simulink model "TST_CoVMD_TrqDesCoord"  (R2016b)
settings: Solver=FixedStepDiscrete  StartTime=0.0  StopTime=simTime  FixedStep=sampleTime  RelTol=1e-3
values from neighbouring files (symbols this model uses):
  testCase = 1    [initTST_CoVMD_TrqDesCoord_001.m]
libraries: simulink x12, UnitTest_Lib x10
settings Model: Creator=zhengjinyan  LastModifiedBy=zhengjinyan
settings DebuggingCC: SignalRangeChecking=error

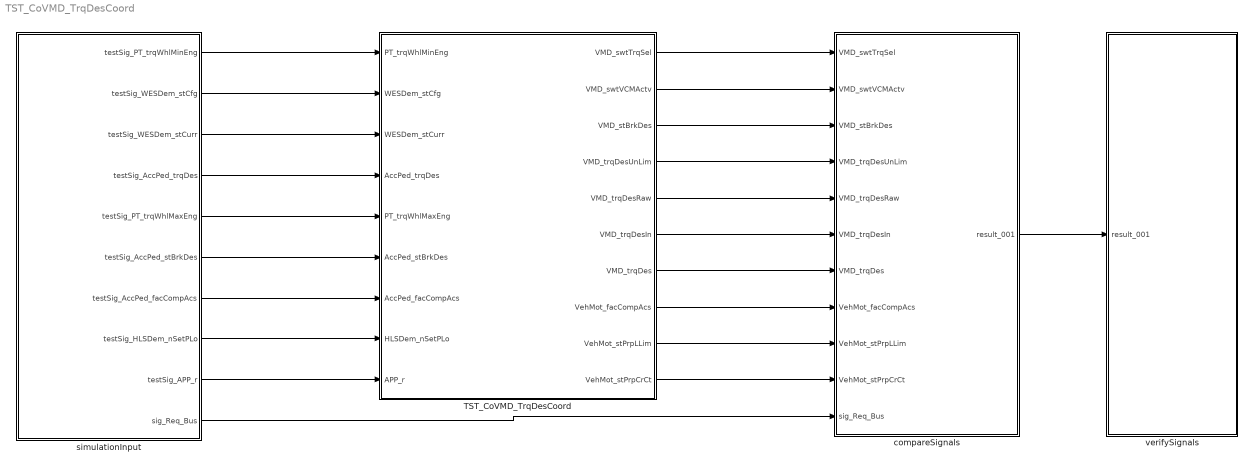
== system TST_CoVMD_TrqDesCoord ==
  TST_CoVMD_TrqDesCoord : Subsystem
  compareSignals : Subsystem
  simulationInput : Subsystem
  verifySignals : Subsystem
  wires:
  simulationInput/1(testSig_PT_trqWhlMinEng) -> TST_CoVMD_TrqDesCoord/1(PT_trqWhlMinEng)
  simulationInput/2(testSig_WESDem_stCfg) -> TST_CoVMD_TrqDesCoord/2(WESDem_stCfg)
  simulationInput/3(testSig_WESDem_stCurr) -> TST_CoVMD_TrqDesCoord/3(WESDem_stCurr)
  simulationInput/4(testSig_AccPed_trqDes) -> TST_CoVMD_TrqDesCoord/4(AccPed_trqDes)
  simulationInput/5(testSig_PT_trqWhlMaxEng) -> TST_CoVMD_TrqDesCoord/5(PT_trqWhlMaxEng)
  simulationInput/6(testSig_AccPed_stBrkDes) -> TST_CoVMD_TrqDesCoord/6(AccPed_stBrkDes)
  simulationInput/7(testSig_AccPed_facCompAcs) -> TST_CoVMD_TrqDesCoord/7(AccPed_facCompAcs)
  simulationInput/8(testSig_HLSDem_nSetPLo) -> TST_CoVMD_TrqDesCoord/8(HLSDem_nSetPLo)
  simulationInput/9(testSig_APP_r) -> TST_CoVMD_TrqDesCoord/9(APP_r)
  TST_CoVMD_TrqDesCoord/1(VMD_swtTrqSel) -> compareSignals/1(VMD_swtTrqSel)
  TST_CoVMD_TrqDesCoord/2(VMD_swtVCMActv) -> compareSignals/2(VMD_swtVCMActv)
  TST_CoVMD_TrqDesCoord/3(VMD_stBrkDes) -> compareSignals/3(VMD_stBrkDes)
  TST_CoVMD_TrqDesCoord/4(VMD_trqDesUnLim) -> compareSignals/4(VMD_trqDesUnLim)
  TST_CoVMD_TrqDesCoord/5(VMD_trqDesRaw) -> compareSignals/5(VMD_trqDesRaw)
  TST_CoVMD_TrqDesCoord/6(VMD_trqDesIn) -> compareSignals/6(VMD_trqDesIn)
  TST_CoVMD_TrqDesCoord/7(VMD_trqDes) -> compareSignals/7(VMD_trqDes)
  TST_CoVMD_TrqDesCoord/8(VehMot_facCompAcs) -> compareSignals/8(VehMot_facCompAcs)
  TST_CoVMD_TrqDesCoord/9(VehMot_stPrpLLim) -> compareSignals/9(VehMot_stPrpLLim)
  TST_CoVMD_TrqDesCoord/10(VehMot_stPrpCrCt) -> compareSignals/10(VehMot_stPrpCrCt)
  simulationInput/10(sig_Req_Bus) -> compareSignals/11(sig_Req_Bus)
  compareSignals/1(result_001) -> verifySignals/1(result_001)

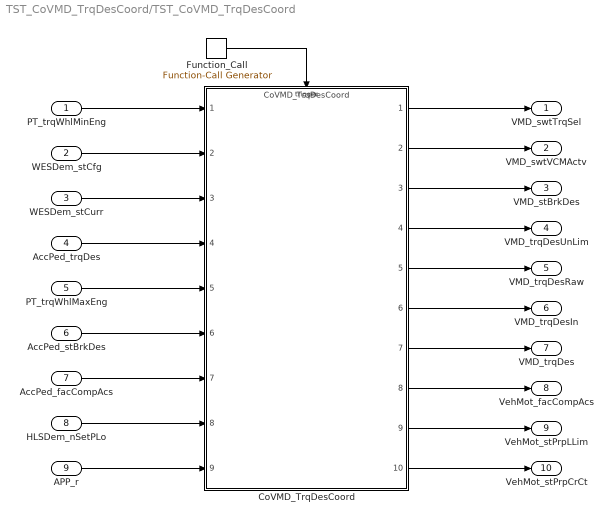
== system TST_CoVMD_TrqDesCoord/TST_CoVMD_TrqDesCoord ==
  PT_trqWhlMinEng : Inport
  WESDem_stCfg : Inport  Port=2
  WESDem_stCurr : Inport  Port=3
  AccPed_trqDes : Inport  Port=4
  PT_trqWhlMaxEng : Inport  Port=5
  AccPed_stBrkDes : Inport  Port=6
  AccPed_facCompAcs : Inport  Port=7
  HLSDem_nSetPLo : Inport  Port=8
  APP_r : Inport  Port=9
  CoVMD_TrqDesCoord : ModelReference  ModelNameDialog=CoVMD_TrqDesCoord  SimulationMode=Normal  ModelReferenceVersion=1.30  TriggerPortName=function  TriggerPortTriggerType=function-call  TriggerPortStatesWhenEnabling=held
  Function_Call : simulink/Ports & Subsystems/Function-Call Generator  sample_time=sampleTime  numberOfIterations=1
  VMD_swtTrqSel : Outport
  VMD_swtVCMActv : Outport  Port=2
  VMD_stBrkDes : Outport  Port=3
  VMD_trqDesUnLim : Outport  Port=4
  VMD_trqDesRaw : Outport  Port=5
  VMD_trqDesIn : Outport  Port=6
  VMD_trqDes : Outport  Port=7
  VehMot_facCompAcs : Outport  Port=8
  VehMot_stPrpLLim : Outport  Port=9
  VehMot_stPrpCrCt : Outport  Port=10
  wires:
  Function_Call/1 -> CoVMD_TrqDesCoord/Trigger
  PT_trqWhlMinEng/1 -> CoVMD_TrqDesCoord/1
  WESDem_stCfg/1 -> CoVMD_TrqDesCoord/2
  WESDem_stCurr/1 -> CoVMD_TrqDesCoord/3
  AccPed_trqDes/1 -> CoVMD_TrqDesCoord/4
  PT_trqWhlMaxEng/1 -> CoVMD_TrqDesCoord/5
  AccPed_stBrkDes/1 -> CoVMD_TrqDesCoord/6
  AccPed_facCompAcs/1 -> CoVMD_TrqDesCoord/7
  HLSDem_nSetPLo/1 -> CoVMD_TrqDesCoord/8
  APP_r/1 -> CoVMD_TrqDesCoord/9
  CoVMD_TrqDesCoord/1 -> VMD_swtTrqSel/1
  CoVMD_TrqDesCoord/2 -> VMD_swtVCMActv/1
  CoVMD_TrqDesCoord/3 -> VMD_stBrkDes/1
  CoVMD_TrqDesCoord/4 -> VMD_trqDesUnLim/1
  CoVMD_TrqDesCoord/5 -> VMD_trqDesRaw/1
  CoVMD_TrqDesCoord/6 -> VMD_trqDesIn/1
  CoVMD_TrqDesCoord/7 -> VMD_trqDes/1
  CoVMD_TrqDesCoord/8 -> VehMot_facCompAcs/1
  CoVMD_TrqDesCoord/9 -> VehMot_stPrpLLim/1
  CoVMD_TrqDesCoord/10 -> VehMot_stPrpCrCt/1

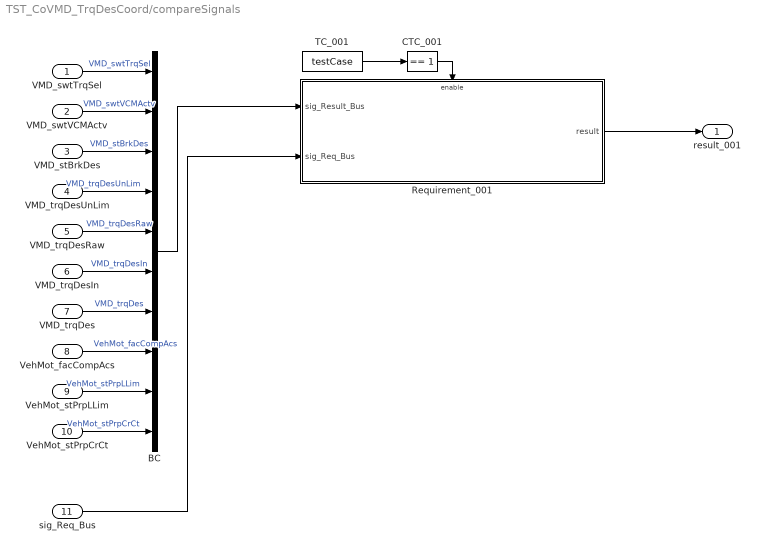
== system TST_CoVMD_TrqDesCoord/compareSignals ==
  VMD_swtTrqSel : Inport
  VMD_swtVCMActv : Inport  Port=2
  VMD_stBrkDes : Inport  Port=3
  VMD_trqDesUnLim : Inport  Port=4
  VMD_trqDesRaw : Inport  Port=5
  VMD_trqDesIn : Inport  Port=6
  VMD_trqDes : Inport  Port=7
  VehMot_facCompAcs : Inport  Port=8
  VehMot_stPrpLLim : Inport  Port=9
  VehMot_stPrpCrCt : Inport  Port=10
  sig_Req_Bus : Inport  Port=11
  BC : BusCreator  Inputs=10
  CTC_001 : simulink/Logic and Bit Operations/Compare To Constant  relop===  const=1  OutDataTypeStr=boolean
  Requirement_001 : Subsystem
  TC_001 : Constant  Value=testCase
  result_001 : Outport
  wires:
  VMD_swtTrqSel/1 -> BC/1  "VMD_swtTrqSel"
  VMD_swtVCMActv/1 -> BC/2  "VMD_swtVCMActv"
  VMD_stBrkDes/1 -> BC/3  "VMD_stBrkDes"
  VMD_trqDesUnLim/1 -> BC/4  "VMD_trqDesUnLim"
  VMD_trqDesRaw/1 -> BC/5  "VMD_trqDesRaw"
  VMD_trqDesIn/1 -> BC/6  "VMD_trqDesIn"
  VMD_trqDes/1 -> BC/7  "VMD_trqDes"
  VehMot_facCompAcs/1 -> BC/8  "VehMot_facCompAcs"
  VehMot_stPrpLLim/1 -> BC/9  "VehMot_stPrpLLim"
  VehMot_stPrpCrCt/1 -> BC/10  "VehMot_stPrpCrCt"
  TC_001/1 -> CTC_001/1
  CTC_001/1 -> Requirement_001/Enable
  sig_Req_Bus/1 -> Requirement_001/2(sig_Req_Bus)
  BC/1 -> Requirement_001/1(sig_Result_Bus)
  Requirement_001/1(result) -> result_001/1

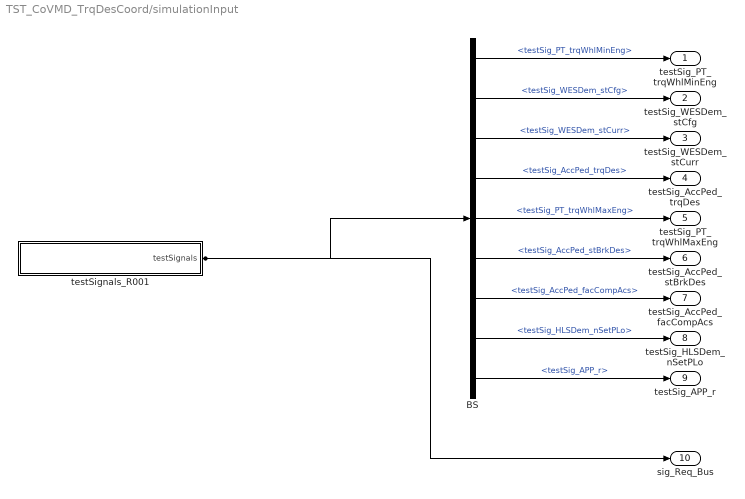
== system TST_CoVMD_TrqDesCoord/simulationInput ==
  BS : BusSelector  OutputSignals=testSig_PT_trqWhlMinEng,testSig_WESDem_stCfg,testSig_WESDem_stCurr,testSig_AccPed_trqDes,testSig_PT_trqWhlMaxEng,testSig_AccPed_stBrkDes,testSig_AccPed_facCompAcs,testSig_HLSDem_nSetPLo,testSig_APP_r
  testSignals_R001 : Subsystem
  testSig_PT_trqWhlMinEng : Outport
  testSig_WESDem_stCfg : Outport  Port=2
  testSig_WESDem_stCurr : Outport  Port=3
  testSig_AccPed_trqDes : Outport  Port=4
  testSig_PT_trqWhlMaxEng : Outport  Port=5
  testSig_AccPed_stBrkDes : Outport  Port=6
  testSig_AccPed_facCompAcs : Outport  Port=7
  testSig_HLSDem_nSetPLo : Outport  Port=8
  testSig_APP_r : Outport  Port=9
  sig_Req_Bus : Outport  Port=10
  wires:
  BS/1 -> testSig_PT_trqWhlMinEng/1  "<testSig_PT_trqWhlMinEng>"
  BS/2 -> testSig_WESDem_stCfg/1  "<testSig_WESDem_stCfg>"
  BS/3 -> testSig_WESDem_stCurr/1  "<testSig_WESDem_stCurr>"
  BS/4 -> testSig_AccPed_trqDes/1  "<testSig_AccPed_trqDes>"
  BS/5 -> testSig_PT_trqWhlMaxEng/1  "<testSig_PT_trqWhlMaxEng>"
  BS/6 -> testSig_AccPed_stBrkDes/1  "<testSig_AccPed_stBrkDes>"
  BS/7 -> testSig_AccPed_facCompAcs/1  "<testSig_AccPed_facCompAcs>"
  BS/8 -> testSig_HLSDem_nSetPLo/1  "<testSig_HLSDem_nSetPLo>"
  BS/9 -> testSig_APP_r/1  "<testSig_APP_r>"
  testSignals_R001/1(testSignals) -> BS/1, sig_Req_Bus/1

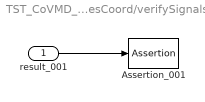
== system TST_CoVMD_TrqDesCoord/verifySignals ==
  result_001 : Inport
  Assertion_001 : Assertion  Enabled=off
  wires:
  result_001/1 -> Assertion_001/1

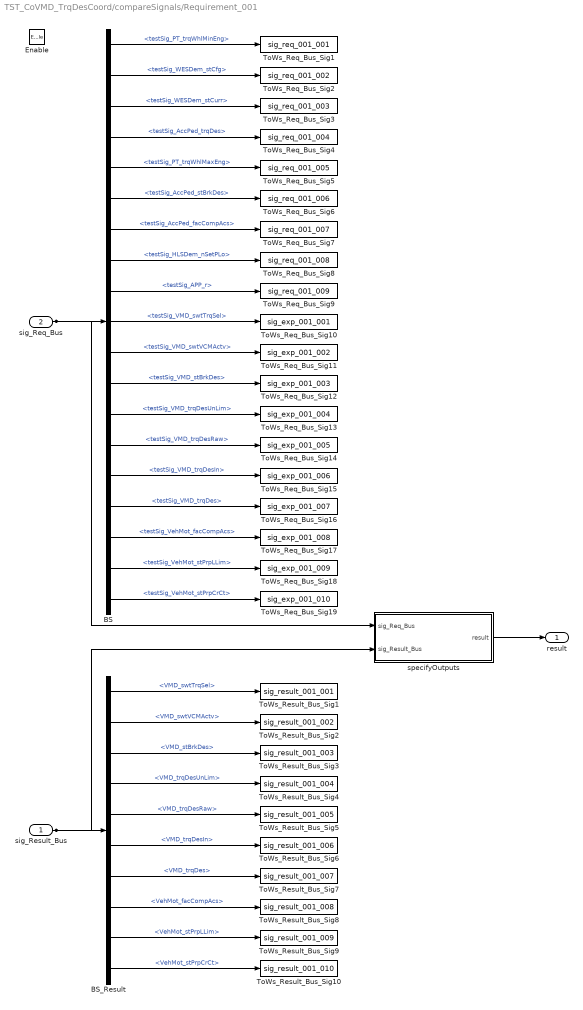
== system TST_CoVMD_TrqDesCoord/compareSignals/Requirement_001 ==
  sig_Result_Bus : Inport
  sig_Req_Bus : Inport  Port=2
  Enable : EnablePort
  BS : BusSelector  OutputSignals=testSig_PT_trqWhlMinEng,testSig_WESDem_stCfg,testSig_WESDem_stCurr,testSig_AccPed_trqDes,testSig_PT_trqWhlMaxEng,testSig_AccPed_stBrkDes,testSig_AccPed_facCompAcs,testSig_HLSDem_nSetPLo,testSig_APP_r,testSig_VMD_swtTrqSel,testSig_VMD_swtVCMActv,testSig_VMD_stBrkDes,testSig_VMD_trqDesUnLim,testSig_VMD_trqDesRaw,testSig_VMD_trqDesIn,testSig_VMD_trqDes,testSig_VehMot_facCompAcs,testSig_VehMot_stPrpLLim,testSig_VehMot_stPrpCrCt
  BS_Result : BusSelector  OutputSignals=VMD_swtTrqSel,VMD_swtVCMActv,VMD_stBrkDes,VMD_trqDesUnLim,VMD_trqDesRaw,VMD_trqDesIn,VMD_trqDes,VehMot_facCompAcs,VehMot_stPrpLLim,VehMot_stPrpCrCt
  ToWs_Req_Bus_Sig1 : ToWorkspace  VariableName=sig_req_001_001  SaveFormat=Structure With Time
  ToWs_Req_Bus_Sig10 : ToWorkspace  VariableName=sig_exp_001_001  SaveFormat=Structure With Time
  ToWs_Req_Bus_Sig11 : ToWorkspace  VariableName=sig_exp_001_002  SaveFormat=Structure With Time
  ToWs_Req_Bus_Sig12 : ToWorkspace  VariableName=sig_exp_001_003  SaveFormat=Structure With Time
  ToWs_Req_Bus_Sig13 : ToWorkspace  VariableName=sig_exp_001_004  SaveFormat=Structure With Time
  ToWs_Req_Bus_Sig14 : ToWorkspace  VariableName=sig_exp_001_005  SaveFormat=Structure With Time
  ToWs_Req_Bus_Sig15 : ToWorkspace  VariableName=sig_exp_001_006  SaveFormat=Structure With Time
  ToWs_Req_Bus_Sig16 : ToWorkspace  VariableName=sig_exp_001_007  SaveFormat=Structure With Time
  ToWs_Req_Bus_Sig17 : ToWorkspace  VariableName=sig_exp_001_008  SaveFormat=Structure With Time
  ToWs_Req_Bus_Sig18 : ToWorkspace  VariableName=sig_exp_001_009  SaveFormat=Structure With Time
  ToWs_Req_Bus_Sig19 : ToWorkspace  VariableName=sig_exp_001_010  SaveFormat=Structure With Time
  ToWs_Req_Bus_Sig2 : ToWorkspace  VariableName=sig_req_001_002  SaveFormat=Structure With Time
  ToWs_Req_Bus_Sig3 : ToWorkspace  VariableName=sig_req_001_003  SaveFormat=Structure With Time
  ToWs_Req_Bus_Sig4 : ToWorkspace  VariableName=sig_req_001_004  SaveFormat=Structure With Time
  ToWs_Req_Bus_Sig5 : ToWorkspace  VariableName=sig_req_001_005  SaveFormat=Structure With Time
  ToWs_Req_Bus_Sig6 : ToWorkspace  VariableName=sig_req_001_006  SaveFormat=Structure With Time
  ToWs_Req_Bus_Sig7 : ToWorkspace  VariableName=sig_req_001_007  SaveFormat=Structure With Time
  ToWs_Req_Bus_Sig8 : ToWorkspace  VariableName=sig_req_001_008  SaveFormat=Structure With Time
  ToWs_Req_Bus_Sig9 : ToWorkspace  VariableName=sig_req_001_009  SaveFormat=Structure With Time
  ToWs_Result_Bus_Sig1 : ToWorkspace  VariableName=sig_result_001_001  SaveFormat=Structure With Time
  ToWs_Result_Bus_Sig10 : ToWorkspace  VariableName=sig_result_001_010  SaveFormat=Structure With Time
  ToWs_Result_Bus_Sig2 : ToWorkspace  VariableName=sig_result_001_002  SaveFormat=Structure With Time
  ToWs_Result_Bus_Sig3 : ToWorkspace  VariableName=sig_result_001_003  SaveFormat=Structure With Time
  ToWs_Result_Bus_Sig4 : ToWorkspace  VariableName=sig_result_001_004  SaveFormat=Structure With Time
  ToWs_Result_Bus_Sig5 : ToWorkspace  VariableName=sig_result_001_005  SaveFormat=Structure With Time
  ToWs_Result_Bus_Sig6 : ToWorkspace  VariableName=sig_result_001_006  SaveFormat=Structure With Time
  ToWs_Result_Bus_Sig7 : ToWorkspace  VariableName=sig_result_001_007  SaveFormat=Structure With Time
  ToWs_Result_Bus_Sig8 : ToWorkspace  VariableName=sig_result_001_008  SaveFormat=Structure With Time
  ToWs_Result_Bus_Sig9 : ToWorkspace  VariableName=sig_result_001_009  SaveFormat=Structure With Time
  specifyOutputs : Subsystem
  result : Outport
  wires:
  sig_Req_Bus/1 -> BS/1, specifyOutputs/1(sig_Req_Bus)
  BS/1 -> ToWs_Req_Bus_Sig1/1  "<testSig_PT_trqWhlMinEng>"
  BS/2 -> ToWs_Req_Bus_Sig2/1  "<testSig_WESDem_stCfg>"
  BS/3 -> ToWs_Req_Bus_Sig3/1  "<testSig_WESDem_stCurr>"
  BS/4 -> ToWs_Req_Bus_Sig4/1  "<testSig_AccPed_trqDes>"
  BS/5 -> ToWs_Req_Bus_Sig5/1  "<testSig_PT_trqWhlMaxEng>"
  BS/6 -> ToWs_Req_Bus_Sig6/1  "<testSig_AccPed_stBrkDes>"
  BS/7 -> ToWs_Req_Bus_Sig7/1  "<testSig_AccPed_facCompAcs>"
  BS/8 -> ToWs_Req_Bus_Sig8/1  "<testSig_HLSDem_nSetPLo>"
  BS/9 -> ToWs_Req_Bus_Sig9/1  "<testSig_APP_r>"
  BS/10 -> ToWs_Req_Bus_Sig10/1  "<testSig_VMD_swtTrqSel>"
  BS/11 -> ToWs_Req_Bus_Sig11/1  "<testSig_VMD_swtVCMActv>"
  BS/12 -> ToWs_Req_Bus_Sig12/1  "<testSig_VMD_stBrkDes>"
  BS/13 -> ToWs_Req_Bus_Sig13/1  "<testSig_VMD_trqDesUnLim>"
  BS/14 -> ToWs_Req_Bus_Sig14/1  "<testSig_VMD_trqDesRaw>"
  BS/15 -> ToWs_Req_Bus_Sig15/1  "<testSig_VMD_trqDesIn>"
  BS/16 -> ToWs_Req_Bus_Sig16/1  "<testSig_VMD_trqDes>"
  BS/17 -> ToWs_Req_Bus_Sig17/1  "<testSig_VehMot_facCompAcs>"
  BS/18 -> ToWs_Req_Bus_Sig18/1  "<testSig_VehMot_stPrpLLim>"
  BS/19 -> ToWs_Req_Bus_Sig19/1  "<testSig_VehMot_stPrpCrCt>"
  sig_Result_Bus/1 -> BS_Result/1, specifyOutputs/2(sig_Result_Bus)
  BS_Result/1 -> ToWs_Result_Bus_Sig1/1  "<VMD_swtTrqSel>"
  BS_Result/2 -> ToWs_Result_Bus_Sig2/1  "<VMD_swtVCMActv>"
  BS_Result/3 -> ToWs_Result_Bus_Sig3/1  "<VMD_stBrkDes>"
  BS_Result/4 -> ToWs_Result_Bus_Sig4/1  "<VMD_trqDesUnLim>"
  BS_Result/5 -> ToWs_Result_Bus_Sig5/1  "<VMD_trqDesRaw>"
  BS_Result/6 -> ToWs_Result_Bus_Sig6/1  "<VMD_trqDesIn>"
  BS_Result/7 -> ToWs_Result_Bus_Sig7/1  "<VMD_trqDes>"
  BS_Result/8 -> ToWs_Result_Bus_Sig8/1  "<VehMot_facCompAcs>"
  BS_Result/9 -> ToWs_Result_Bus_Sig9/1  "<VehMot_stPrpLLim>"
  BS_Result/10 -> ToWs_Result_Bus_Sig10/1  "<VehMot_stPrpCrCt>"
  specifyOutputs/1(result) -> result/1

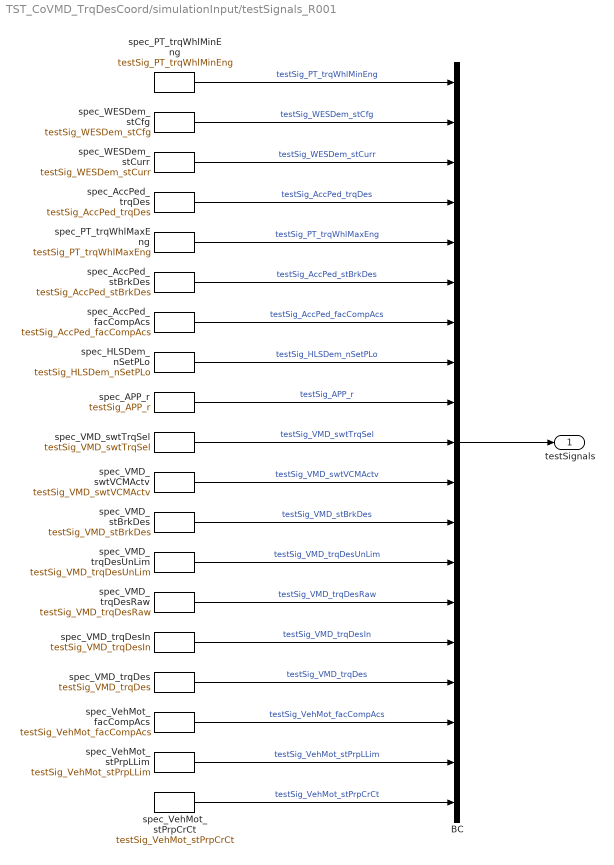
== system TST_CoVMD_TrqDesCoord/simulationInput/testSignals_R001 ==
  BC : BusCreator  Inputs=19
  spec_APP_r : FromWorkspace  VariableName=testSig_APP_r  Interpolate=off  OutputAfterFinalValue=Holding final value
  spec_AccPed_facCompAcs : FromWorkspace  VariableName=testSig_AccPed_facCompAcs  Interpolate=off  OutputAfterFinalValue=Holding final value
  spec_AccPed_stBrkDes : FromWorkspace  VariableName=testSig_AccPed_stBrkDes  Interpolate=off  OutputAfterFinalValue=Holding final value
  spec_AccPed_trqDes : FromWorkspace  VariableName=testSig_AccPed_trqDes  Interpolate=off  OutputAfterFinalValue=Holding final value
  spec_HLSDem_nSetPLo : FromWorkspace  VariableName=testSig_HLSDem_nSetPLo  Interpolate=off  OutputAfterFinalValue=Holding final value
  spec_PT_trqWhlMaxEng : FromWorkspace  VariableName=testSig_PT_trqWhlMaxEng  Interpolate=off  OutputAfterFinalValue=Holding final value
  spec_PT_trqWhlMinEng : FromWorkspace  VariableName=testSig_PT_trqWhlMinEng  Interpolate=off  OutputAfterFinalValue=Holding final value
  spec_VMD_stBrkDes : FromWorkspace  VariableName=testSig_VMD_stBrkDes  Interpolate=off  OutputAfterFinalValue=Holding final value
  spec_VMD_swtTrqSel : FromWorkspace  VariableName=testSig_VMD_swtTrqSel  Interpolate=off  OutputAfterFinalValue=Holding final value
  spec_VMD_swtVCMActv : FromWorkspace  VariableName=testSig_VMD_swtVCMActv  Interpolate=off  OutputAfterFinalValue=Holding final value
  spec_VMD_trqDes : FromWorkspace  VariableName=testSig_VMD_trqDes  Interpolate=off  OutputAfterFinalValue=Holding final value
  spec_VMD_trqDesIn : FromWorkspace  VariableName=testSig_VMD_trqDesIn  Interpolate=off  OutputAfterFinalValue=Holding final value
  spec_VMD_trqDesRaw : FromWorkspace  VariableName=testSig_VMD_trqDesRaw  Interpolate=off  OutputAfterFinalValue=Holding final value
  spec_VMD_trqDesUnLim : FromWorkspace  VariableName=testSig_VMD_trqDesUnLim  Interpolate=off  OutputAfterFinalValue=Holding final value
  spec_VehMot_facCompAcs : FromWorkspace  VariableName=testSig_VehMot_facCompAcs  Interpolate=off  OutputAfterFinalValue=Holding final value
  spec_VehMot_stPrpCrCt : FromWorkspace  VariableName=testSig_VehMot_stPrpCrCt  Interpolate=off  OutputAfterFinalValue=Holding final value
  spec_VehMot_stPrpLLim : FromWorkspace  VariableName=testSig_VehMot_stPrpLLim  Interpolate=off  OutputAfterFinalValue=Holding final value
  spec_WESDem_stCfg : FromWorkspace  VariableName=testSig_WESDem_stCfg  Interpolate=off  OutputAfterFinalValue=Holding final value
  spec_WESDem_stCurr : FromWorkspace  VariableName=testSig_WESDem_stCurr  Interpolate=off  OutputAfterFinalValue=Holding final value
  testSignals : Outport
  wires:
  BC/1 -> testSignals/1
  spec_PT_trqWhlMinEng/1 -> BC/1  "testSig_PT_trqWhlMinEng"
  spec_WESDem_stCfg/1 -> BC/2  "testSig_WESDem_stCfg"
  spec_WESDem_stCurr/1 -> BC/3  "testSig_WESDem_stCurr"
  spec_AccPed_trqDes/1 -> BC/4  "testSig_AccPed_trqDes"
  spec_PT_trqWhlMaxEng/1 -> BC/5  "testSig_PT_trqWhlMaxEng"
  spec_AccPed_stBrkDes/1 -> BC/6  "testSig_AccPed_stBrkDes"
  spec_AccPed_facCompAcs/1 -> BC/7  "testSig_AccPed_facCompAcs"
  spec_HLSDem_nSetPLo/1 -> BC/8  "testSig_HLSDem_nSetPLo"
  spec_APP_r/1 -> BC/9  "testSig_APP_r"
  spec_VMD_swtTrqSel/1 -> BC/10  "testSig_VMD_swtTrqSel"
  spec_VMD_swtVCMActv/1 -> BC/11  "testSig_VMD_swtVCMActv"
  spec_VMD_stBrkDes/1 -> BC/12  "testSig_VMD_stBrkDes"
  spec_VMD_trqDesUnLim/1 -> BC/13  "testSig_VMD_trqDesUnLim"
  spec_VMD_trqDesRaw/1 -> BC/14  "testSig_VMD_trqDesRaw"
  spec_VMD_trqDesIn/1 -> BC/15  "testSig_VMD_trqDesIn"
  spec_VMD_trqDes/1 -> BC/16  "testSig_VMD_trqDes"
  spec_VehMot_facCompAcs/1 -> BC/17  "testSig_VehMot_facCompAcs"
  spec_VehMot_stPrpLLim/1 -> BC/18  "testSig_VehMot_stPrpLLim"
  spec_VehMot_stPrpCrCt/1 -> BC/19  "testSig_VehMot_stPrpCrCt"

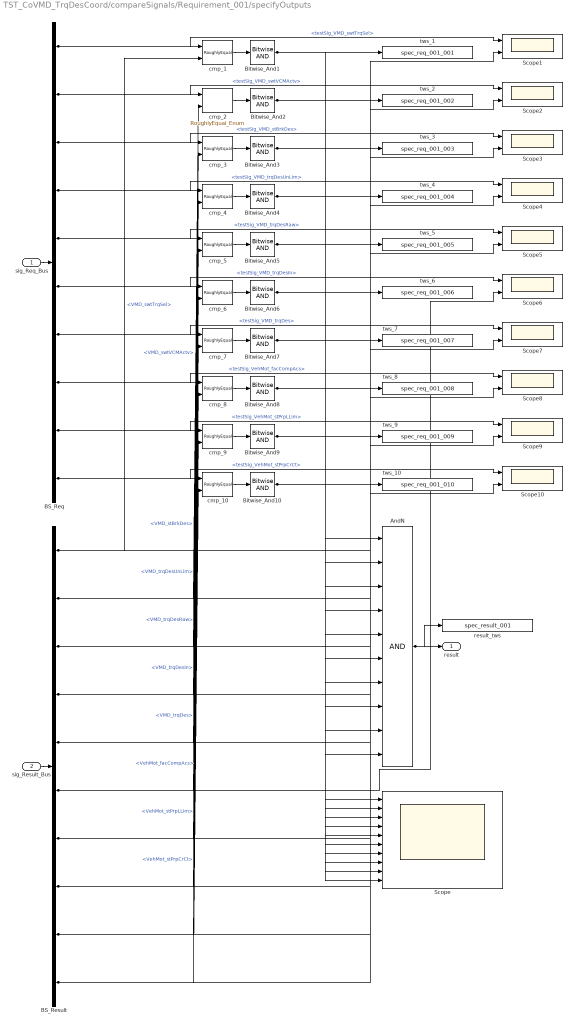
== system TST_CoVMD_TrqDesCoord/compareSignals/Requirement_001/specifyOutputs ==
  sig_Req_Bus : Inport
  sig_Result_Bus : Inport  Port=2
  AndN : Logic  Inputs=10
  BS_Req : BusSelector  OutputSignals=testSig_VMD_swtTrqSel,testSig_VMD_swtVCMActv,testSig_VMD_stBrkDes,testSig_VMD_trqDesUnLim,testSig_VMD_trqDesRaw,testSig_VMD_trqDesIn,testSig_VMD_trqDes,testSig_VehMot_facCompAcs,testSig_VehMot_stPrpLLim,testSig_VehMot_stPrpCrCt
  BS_Result : BusSelector  OutputSignals=VMD_swtTrqSel,VMD_swtVCMActv,VMD_stBrkDes,VMD_trqDesUnLim,VMD_trqDesRaw,VMD_trqDesIn,VMD_trqDes,VehMot_facCompAcs,VehMot_stPrpLLim,VehMot_stPrpCrCt
  Bitwise_And{1..10} (10 alike) : simulink/Logic and Bit Operations/Bitwise Operator  logicop=AND  UseBitMask=off  BitMask=bin2dec('11011001')  BitMaskRealWorld=Stored Integer
  Scope : Scope  NumInputPorts=10
  Scope{1..10} (10 alike) : Scope  NumInputPorts=2
  cmp_{1,3..10} (9 alike) : UnitTest_Lib/RoughlyEqual  slope=0.1
  cmp_2 : UnitTest_Lib/RoughlyEqual_Enum  slope=0.1
  result_tws : ToWorkspace  VariableName=spec_result_001
  tws_1 : ToWorkspace  VariableName=spec_req_001_001
  tws_10 : ToWorkspace  VariableName=spec_req_001_010
  tws_2 : ToWorkspace  VariableName=spec_req_001_002
  tws_3 : ToWorkspace  VariableName=spec_req_001_003
  tws_4 : ToWorkspace  VariableName=spec_req_001_004
  tws_5 : ToWorkspace  VariableName=spec_req_001_005
  tws_6 : ToWorkspace  VariableName=spec_req_001_006
  tws_7 : ToWorkspace  VariableName=spec_req_001_007
  tws_8 : ToWorkspace  VariableName=spec_req_001_008
  tws_9 : ToWorkspace  VariableName=spec_req_001_009
  result : Outport
  wires:
  sig_Req_Bus/1 -> BS_Req/1
  sig_Result_Bus/1 -> BS_Result/1
  AndN/1 -> result/1, result_tws/1
  BS_Req/1 -> cmp_1/1, Scope1/1  "<testSig_VMD_swtTrqSel>"
  BS_Result/1 -> cmp_1/2, Scope1/2  "<VMD_swtTrqSel>"
  cmp_1/1 -> Bitwise_And1/1
  Bitwise_And1/1 -> tws_1/1, AndN/1, Scope/1
  BS_Req/2 -> cmp_2/1, Scope2/1  "<testSig_VMD_swtVCMActv>"
  BS_Result/2 -> cmp_2/2, Scope2/2  "<VMD_swtVCMActv>"
  cmp_2/1 -> Bitwise_And2/1
  Bitwise_And2/1 -> tws_2/1, AndN/2, Scope/2
  BS_Req/3 -> cmp_3/1, Scope3/1  "<testSig_VMD_stBrkDes>"
  BS_Result/3 -> cmp_3/2, Scope3/2  "<VMD_stBrkDes>"
  cmp_3/1 -> Bitwise_And3/1
  Bitwise_And3/1 -> tws_3/1, AndN/3, Scope/3
  BS_Req/4 -> cmp_4/1, Scope4/1  "<testSig_VMD_trqDesUnLim>"
  BS_Result/4 -> cmp_4/2, Scope4/2  "<VMD_trqDesUnLim>"
  cmp_4/1 -> Bitwise_And4/1
  Bitwise_And4/1 -> tws_4/1, AndN/4, Scope/4
  BS_Req/5 -> cmp_5/1, Scope5/1  "<testSig_VMD_trqDesRaw>"
  BS_Result/5 -> cmp_5/2, Scope5/2  "<VMD_trqDesRaw>"
  cmp_5/1 -> Bitwise_And5/1
  Bitwise_And5/1 -> tws_5/1, AndN/5, Scope/5
  BS_Req/6 -> cmp_6/1, Scope6/1  "<testSig_VMD_trqDesIn>"
  BS_Result/6 -> cmp_6/2, Scope6/2  "<VMD_trqDesIn>"
  cmp_6/1 -> Bitwise_And6/1
  Bitwise_And6/1 -> tws_6/1, AndN/6, Scope/6
  BS_Req/7 -> cmp_7/1, Scope7/1  "<testSig_VMD_trqDes>"
  BS_Result/7 -> cmp_7/2, Scope7/2  "<VMD_trqDes>"
  cmp_7/1 -> Bitwise_And7/1
  Bitwise_And7/1 -> tws_7/1, AndN/7, Scope/7
  BS_Req/8 -> cmp_8/1, Scope8/1  "<testSig_VehMot_facCompAcs>"
  BS_Result/8 -> cmp_8/2, Scope8/2  "<VehMot_facCompAcs>"
  cmp_8/1 -> Bitwise_And8/1
  Bitwise_And8/1 -> tws_8/1, AndN/8, Scope/8
  BS_Req/9 -> cmp_9/1, Scope9/1  "<testSig_VehMot_stPrpLLim>"
  BS_Result/9 -> cmp_9/2, Scope9/2  "<VehMot_stPrpLLim>"
  cmp_9/1 -> Bitwise_And9/1
  Bitwise_And9/1 -> tws_9/1, AndN/9, Scope/9
  BS_Req/10 -> cmp_10/1, Scope10/1  "<testSig_VehMot_stPrpCrCt>"
  BS_Result/10 -> cmp_10/2, Scope10/2  "<VehMot_stPrpCrCt>"
  cmp_10/1 -> Bitwise_And10/1
  Bitwise_And10/1 -> tws_10/1, AndN/10, Scope/10
